simulink model "ctrl_2x2"  (Simulink 7.9)
settings: Solver=FixedStepDiscrete  StartTime=0.0  StopTime=tend  FixedStep=params.th  MaxStep=0.01  RelTol=1e-6  AbsTol=1e-3
values from neighbouring files (symbols this model uses):
  amp_DeltaT1 = 0    [ctrl_design.m]    (also in ctrl_design_v2.m)
  amp_DeltaT2 = 0    [ctrl_design.m]    (also in ctrl_design_v2.m)
  delta_cp = 0    [ctrl_design.m]    (also in ctrl_design_v2.m)
  delta_k = 12    [ctrl_design.m]    (also in ctrl_design_v2.m)
  enable_ctrl_pot = 1    [ctrl_design.m]    (also in ctrl_design_v2.m)
  enable_ctrl_vel = 1    [ctrl_design.m]    (also in ctrl_design_v2.m)
  Gc_pot_d = c2d(Gc_pot,params.th,'tustin')    [ctrl_design.m]    (also in ctrl_design_v2.m)
  Gc_vel_d = c2d(Gc_vel,params.th,'tustin')    [ctrl_design.m]    (also in ctrl_design_v2.m)
  t_step_cp = 0    [ctrl_design.m]    (also in ctrl_design_v2.m)
  t_step_k = 5    [ctrl_design.m]    (also in ctrl_design_v2.m)
  t_step_T1 = 0    [ctrl_design.m]    (also in ctrl_design_v2.m)
  t_step_T2 = 0    [ctrl_design.m]    (also in ctrl_design_v2.m)
undefined symbols (not defined in the file or in its folder): params
settings Model: Creator=puri  LastModifiedBy=jorge.elso
settings CodeAppCC: CustomSymbolStrType=$N$R$M_T
settings GRTTargetCC: CodeReplacementLibrary=None  CPPClassGenCompliant=on

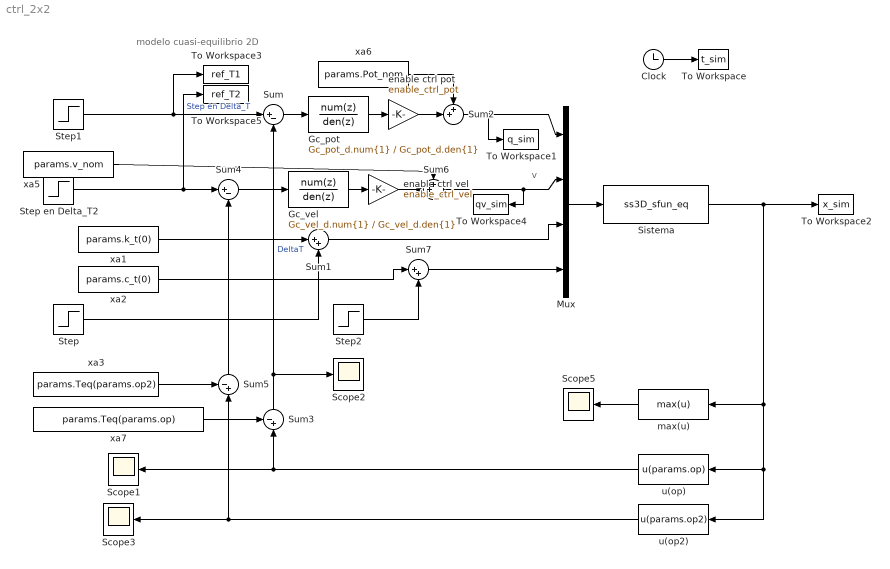
== system ctrl_2x2 ==
  note: modelo cuasi-equilibrio 2D
  note: v
  Clock : Clock
  Gc_pot : DiscreteTransferFcn  Numerator=Gc_pot_d.num{1}  Denominator=Gc_pot_d.den{1}  SampleTime=params.th
  Gc_vel : DiscreteTransferFcn  Numerator=Gc_vel_d.num{1}  Denominator=Gc_vel_d.den{1}  SampleTime=params.th
  Mux : Mux
  Scope{1..3,5} (4 alike) : Scope
      Scope1 settings: TimeRange=4  YMin=1204.12  YMax=1330.86
      Scope2 settings: TimeRange=4  YMin=-1.43245e-12  YMax=-1.29603e-12
      Scope3 settings: TimeRange=4  YMin=1204.12  YMax=1330.86  SaveName=ScopeData2
      Scope5 settings: TimeRange=4  YMin=4942.75  YMax=4948  SaveName=ScopeData5
  Sistema : S-Function  FunctionName=ss3D_sfun_eq  EnableBusSupport=off
      settings: DeleteFcn=shh = get(0,'ShowHiddenHandles');set(0,'ShowHiddenHandles','on');if ~isempty(findobj('type','figure','name','dblcart1 Animation'));close('dblcart1 Animation'); end;set(0,'ShowHiddenHandles',shh);
  Step : Step  Time=t_step_k  After=delta_k  SampleTime=0
  Step en Delta_T2 : Step  Time=t_step_T2  After=amp_DeltaT2  SampleTime=0
  Step1 : Step  Time=t_step_T1  After=amp_DeltaT1  SampleTime=0
  Step2 : Step  Time=t_step_cp  After=delta_cp  SampleTime=0
  Sum : Sum  Inputs=|+-
  Sum1 : Sum  Inputs=|++
  Sum2 : Sum  Inputs=++|
  Sum3 : Sum  Inputs=-+|
  Sum4 : Sum  Inputs=|+-
  Sum5 : Sum  Inputs=-+|
  Sum6 : Sum  Inputs=++|
  Sum7 : Sum  Inputs=|++
  To Workspace : ToWorkspace  VariableName=t_sim  SampleTime=-1
  To Workspace1 : ToWorkspace  VariableName=q_sim  SampleTime=-1
  To Workspace2 : ToWorkspace  VariableName=x_sim  SampleTime=-1
  To Workspace3 : ToWorkspace  VariableName=ref_T1  SampleTime=-1
  To Workspace4 : ToWorkspace  VariableName=qv_sim  SampleTime=-1
  To Workspace5 : ToWorkspace  VariableName=ref_T2  SampleTime=-1
  enable ctrl pot : Gain  Gain=enable_ctrl_pot
  enable ctrl vel : Gain  Gain=enable_ctrl_vel
  max(u) : MATLABFcn  MATLABFcn=max(u)
  u(op) : MATLABFcn  MATLABFcn=u(params.op)
  u(op2) : MATLABFcn  MATLABFcn=u(params.op2)
  xa1 : Constant  Value=params.k_t(0)
  xa2 : Constant  Value=params.c_t(0)
  xa3 : Constant  Value=params.Teq(params.op2)
  xa5 : Constant  Value=params.v_nom
  xa6 : Constant  Value=params.Pot_nom
  xa7 : Constant  Value=params.Teq(params.op)
  wires:
  Mux/1 -> Sistema/1
  Sistema/1 -> To Workspace2/1, max(u)/1, u(op)/1, u(op2)/1
  Clock/1 -> To Workspace/1
  max(u)/1 -> Scope5/1
  u(op)/1 -> Scope1/1, Sum3/2
  Sum/1 -> Gc_pot/1
  xa1/1 -> Sum1/1
  Sum1/1 -> Mux/3
  Step/1 -> Sum1/2
  Sum2/1 -> To Workspace1/1, Mux/1
  xa6/1 -> Sum2/1
  xa7/1 -> Sum3/1
  Sum3/1 -> Sum/2, Scope2/1  "DeltaT"
  Step1/1 -> Sum/1, To Workspace3/1  "Step en Delta_T"
  Gc_pot/1 -> enable ctrl pot/1
  xa3/1 -> Sum5/1
  Step en Delta_T2/1 -> Sum4/1, To Workspace5/1
  Sum5/1 -> Sum4/2
  Sum4/1 -> Gc_vel/1
  xa5/1 -> Sum6/1
  Gc_vel/1 -> enable ctrl vel/1
  u(op2)/1 -> Scope3/1, Sum5/2
  Sum6/1 -> To Workspace4/1, Mux/2
  enable ctrl vel/1 -> Sum6/2
  enable ctrl pot/1 -> Sum2/2
  Sum7/1 -> Mux/4
  xa2/1 -> Sum7/1
  Step2/1 -> Sum7/2
